simulink library "sensors_lib"  (R2016b)
settings: Solver=ode45  StartTime=0.0  StopTime=10.0  RelTol=1e-3  EnableMultiTasking=on
undefined symbols (not defined in the file or in its folder): GPS, mag_eci_T, measurements_deg_err, measurements_valid, omega_radps_gyro, sun_eci_unit_photodiode, sun_eci_unit_sunsensor
libraries: gps x1, bus_stubs_template x1, gyroscope_lib x1, magnetometer_lib x1, photodiodes_lib x1, sun_sensor_lib x1
settings Model: Creator=bbarz_000  LastModifiedBy=taylorreynolds
settings DataIOCC: LimitDataPoints=on
settings OptimizationCC: LifeSpan=inf
settings DebuggingCC: AllowSymbolicDim=off  SFUnexpectedBacktrackingDiag=warning  SFNoUnconditionalDefaultTransitionDiag=warning  SFExecutionAtInitializationDiag=none
settings GRTTargetCC: TargetLangStandard=C89/C90 (ANSI)  GeneratePreprocessorConditionals=Disable all
settings ConfigComp: CovMetricSettings=dw  CovHtmlReporting=on  CovSaveCumulativeToWorkspaceVar=on  CovSaveSingleToWorkspaceVar=on  CovExternalEMLEnable=off

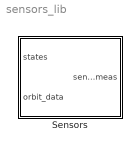
== system sensors_lib ==
  Sensors : Subsystem

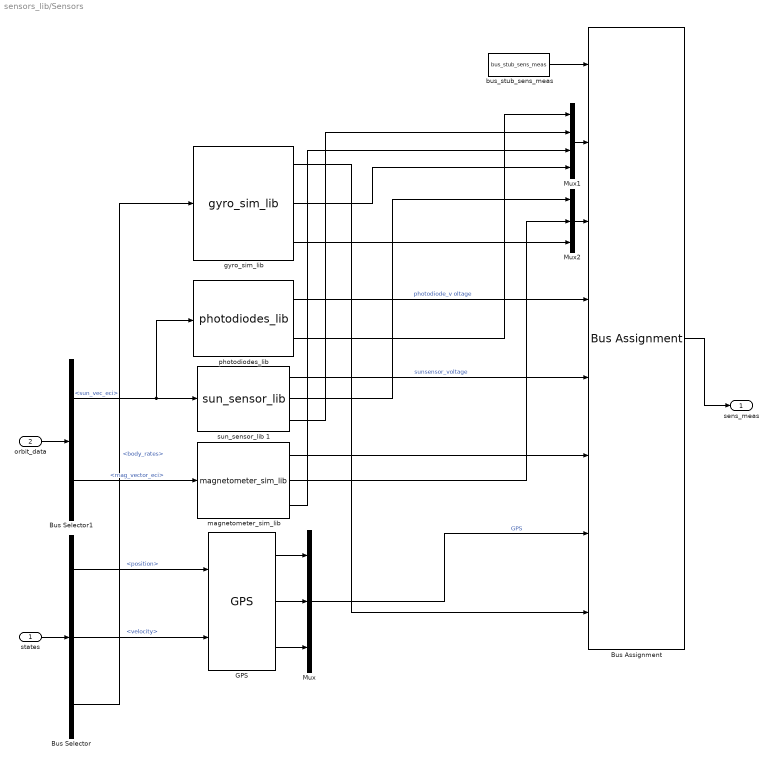
== system sensors_lib/Sensors ==
  states : Inport  OutDataTypeStr=Bus: states
  orbit_data : Inport  Port=2  OutDataTypeStr=Bus: orbit_data
  Bus Assignment : BusAssignment  AssignedSignals=measurements_deg_err,measurements_valid,sun_eci_unit_photodiode,sun_eci_unit_sunsensor,mag_eci_T,GPS,omega_radps_gyro
  Bus Selector : BusSelector  OutputSignals=position,velocity,body_rates
  Bus Selector1 : BusSelector  OutputSignals=sun_vec_eci,mag_vector_eci
  GPS : gps/GPS
  Mux : Mux  Inputs=[3 3 2]
  Mux1 : Mux
  Mux2 : Mux  Inputs=3
  bus_stub_sens_meas : bus_stubs_template/bus_stub_sens_meas
  gyro_sim_lib : gyroscope_lib/gyro_sim_lib
  magnetometer_sim_lib : magnetometer_lib/magnetometer_sim_lib
  photodiodes_lib : photodiodes_lib/photodiodes_lib
  sun_sensor_lib 1 : sun_sensor_lib/sun_sensor_lib 
  sens_meas : Outport
  wires:
  states/1 -> Bus Selector/1
  Bus Assignment/1 -> sens_meas/1
  photodiodes_lib/1 -> Bus Assignment/4  "photodiode_v oltage"
  sun_sensor_lib 1/1 -> Bus Assignment/5  "sunsensor_voltage"
  Mux/1 -> Bus Assignment/7  "GPS"
  bus_stub_sens_meas/1 -> Bus Assignment/1
  Bus Selector/3 -> gyro_sim_lib/1  "<body_rates>"
  orbit_data/1 -> Bus Selector1/1
  gyro_sim_lib/1 -> Bus Assignment/8
  Bus Selector/2 -> GPS/2  "<velocity>"
  Bus Selector/1 -> GPS/1  "<position>"
  GPS/1 -> Mux/1
  GPS/2 -> Mux/2
  magnetometer_sim_lib/1 -> Bus Assignment/6
  Bus Selector1/2 -> magnetometer_sim_lib/1  "<mag_vector_eci>"
  Bus Selector1/1 -> sun_sensor_lib 1/1, photodiodes_lib/1  "<sun_vec_eci>"
  GPS/3 -> Mux/3
  Mux1/1 -> Bus Assignment/2
  photodiodes_lib/2 -> Mux1/1
  sun_sensor_lib 1/3 -> Mux1/2
  magnetometer_sim_lib/3 -> Mux1/3
  gyro_sim_lib/2 -> Mux1/4
  Mux2/1 -> Bus Assignment/3
  gyro_sim_lib/3 -> Mux2/3
  magnetometer_sim_lib/2 -> Mux2/2
  sun_sensor_lib 1/2 -> Mux2/1
